simulink library "etherlab_lib_exp"  (Simulink 6.4)
undefined symbols (not defined in the file or in its folder): Address, catch_check
(part 3 of 3)

== system etherlab_lib_exp/Generate Code ==

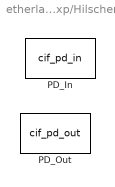
== system etherlab_lib_exp/Hilscher ==
  PD_In : S-Function  FunctionName=cif_pd_in  Parameters=device,addr,ip_type,width,swap,op_type,tsample  mask(Profibus Input){device=01:0E, addr=120, ip_type=int8_T, width=8, swap=off, op_type=int8, tsample=0}
      mask prompts: device "PCI Device"; addr "Address"; ip_type "Sensor Data Type"; width "Vector Length"; swap "Swap Input Bytes"; op_type "Output Data Format"; tsample "Sample Time (-1 inherited)"
      mask help: Hilscher CIF-80PB Profibus Input
      mask init:
      | device = test_var(device);
      mask Help:
      | This block provides an interface to the Profibus incoming process image for the Hilscher CIF-80PB Card.
      | <p>
      | Supply the following information:<br>
      | <b>PCI Device</b>: Either supply the address in PCI-Addressing format <em>bus:slot</em> (hexadecimal format), or the (decimal) position as cards are detected
      mask StyleString: edit,edit,popup(Bit0|Bit1|Bit2|Bit3|Bit4|Bit5|Bit6 |Bit7|int8_T|uint8_T|int16_T|uint16_T|int32_T|uint32_T),edit,checkbox,popup(int8|uint8|int16|uint16|int32|uint32|boolean|double|single|Inherited via back propagation),edit
      mask Display:
      | fprintf('CIF-80PB\nPCI: %s\nAddr:%i',
      | device,addr);
  PD_Out : S-Function  FunctionName=cif_pd_out  Parameters=device,addr,op_type,swap,tsample  mask(Profibus Input){device=01:0E, addr=120, op_type=int8_T, swap=off, tsample=-1}
      mask prompts: device "PCI Device"; addr "Address"; op_type "Actuator Data Type"; swap "Swap Input Bytes"; tsample "Sample Time (-1 inherited)"
      mask help: Hilscher CIF-80PB Profibus Output
      mask init:
      | device = test_var(device);
      mask Help:
      | This block provides an interface to the Profibus outgoing process image for the Hilscher CIF-80PB Card.
      | <p>
      | Supply the following information:<br>
      | <b>PCI Device</b>: Either supply the address in PCI-Addressing format <em>bus:slot</em> (hexadecimal format), or the (decimal) position as cards are detected
      mask StyleString: edit,edit,popup(Bit0|Bit1|Bit2|Bit3|Bit4|Bit5|Bit6 |Bit7|int8_T|uint8_T|int16_T|uint16_T|int32_T|uint32_T),checkbox,edit
      mask Display:
      | fprintf('CIF-80PB\nPCI: %s\nAddr:%i',
      | device,addr);

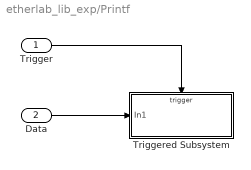
== system etherlab_lib_exp/Printf ==
  Trigger : Inport
  Data : Inport  Port=2
  Triggered Subsystem : Subsystem  TreatAsAtomicUnit=on
  wires:
  Trigger/1 -> Triggered Subsystem/Trigger
  Data/1 -> Triggered Subsystem/1(In1)

== system etherlab_lib_exp/cbdb ==

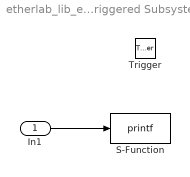
== system etherlab_lib_exp/Printf/Triggered Subsystem ==
  In1 : Inport
  Trigger : TriggerPort
  S-Function : S-Function  FunctionName=printf  Parameters=format
  wires:
  In1/1 -> S-Function/1
